simulink model "delay"  (R2025b)
settings: Solver=FixedStepDiscrete  StartTime=0.0  StopTime=inf  RelTol=1e-3
model workspace (MATLAB code in the model file):
  | Mix_rt = Simulink.Parameter(0.50);
  | Mix_rt.CoderInfo.StorageClass = 'Auto';   % <- NO ExportedGlobal
undefined symbols (not defined in the file): Mode_rt, Repeats_rt, Time_rt
settings Model: Creator=linogarciamorales  LastModifiedBy=linogarciamorales
settings OptimizationCC: EnhancedBackFolding=on  PassReuseOutputArgsAs=Individual arguments  ZeroExternalMemoryAtStartup=off  ZeroInternalMemoryAtStartup=off  OptimizeBlockOrder=speed  DifferentSizesBufferReuse=on  OptimizationCustomize=off  EfficientTunableParamExpr=on
settings DebuggingCC: ParameterTunabilityLossMsg=error
settings SFSimCC: MATLABDynamicMemAlloc=off
settings RTWCC: SystemTargetFile=ert.tlc  GenCodeOnly=on  TemplateMakefile=ert_default_tmf  Description=Embedded Coder
settings CodeAppCC: ForceParamTrailComments=on  IgnoreCustomStorageClasses=off  OperatorAnnotations=on  SimulinkDataObjDesc=on  SFDataObjDesc=on  InsertBlockDesc=on
settings ERTTargetCC: InlinedParameterPlacement=Hierarchical  ERTCustomFileTemplate=example_file_process.tlc  TargetLangStandard=C99 (ISO)  GenerateSampleERTMain=on  SupportNonInlinedSFcns=on

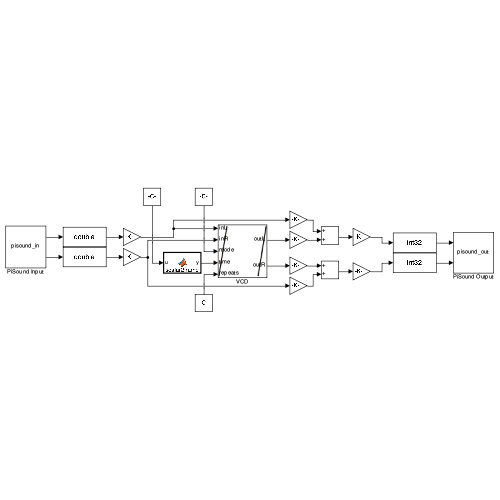
[thumbnail: Simulink's stored preview of the top-level diagram]
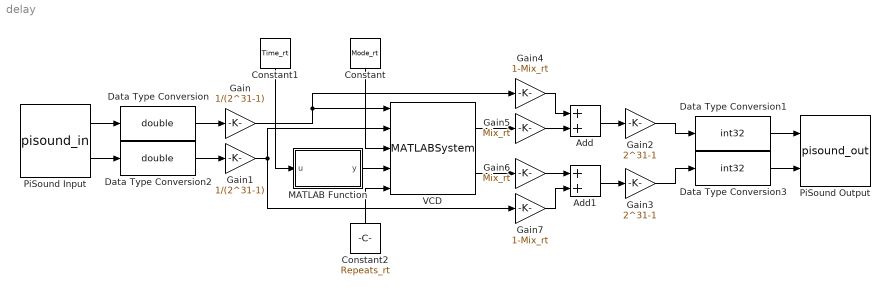
== system delay ==
  Add : Sum
  Add1 : Sum
  Constant : Constant  Value=Mode_rt  OutDataTypeStr=uint8
  Constant1 : Constant  Value=Time_rt  OutDataTypeStr=double
  Constant2 : Constant  Value=Repeats_rt  OutDataTypeStr=double
  Data Type Conversion : DataTypeConversion  OutDataTypeStr=double  SaturateOnIntegerOverflow=off  RndMeth=Floor
  Data Type Conversion1 : DataTypeConversion  OutDataTypeStr=int32  SaturateOnIntegerOverflow=off  RndMeth=Floor
  Data Type Conversion2 : DataTypeConversion  OutDataTypeStr=double  SaturateOnIntegerOverflow=off  RndMeth=Floor
  Data Type Conversion3 : DataTypeConversion  OutDataTypeStr=int32  SaturateOnIntegerOverflow=off  RndMeth=Floor
  Gain : Gain  Gain=1/(2^31-1)
  Gain1 : Gain  Gain=1/(2^31-1)
  Gain2 : Gain  Gain=2^31-1
  Gain3 : Gain  Gain=2^31-1
  Gain4 : Gain  Gain=1-Mix_rt  OutDataTypeStr=double
  Gain5 : Gain  Gain=Mix_rt  OutDataTypeStr=double
  Gain6 : Gain  Gain=Mix_rt  OutDataTypeStr=double
  Gain7 : Gain  Gain=1-Mix_rt  OutDataTypeStr=double
  MATLAB Function : MATLAB Function  TreatAsAtomicUnit=on
  PiSound Input : S-Function  FunctionName=pisound_in  Parameters=48000, 128, 0  SFunctionDeploymentMode=off  EnableBusSupport=off
  PiSound Output : S-Function  FunctionName=pisound_out  Parameters=48000, 128, 0  SFunctionDeploymentMode=off  EnableBusSupport=off
  VCD : MATLABSystem  System=vcd_sys  N=128  Fs=48000  MaxDelay=2  Mode=uint8(1)  Delay=0.1  g=0.5  SimulateUsing=Code generation
      mask Type: vcd_sys
  wires:
  PiSound Input/1 -> Data Type Conversion/1
  PiSound Input/2 -> Data Type Conversion2/1
  Data Type Conversion1/1 -> PiSound Output/1
  Data Type Conversion3/1 -> PiSound Output/2
  Gain2/1 -> Data Type Conversion1/1
  Gain3/1 -> Data Type Conversion3/1
  Data Type Conversion/1 -> Gain/1
  Data Type Conversion2/1 -> Gain1/1
  Gain/1 -> Gain4/1, VCD/1
  Gain1/1 -> Gain7/1, VCD/2
  VCD/1 -> Gain5/1
  VCD/2 -> Gain6/1
  Constant/1 -> VCD/3
  Constant2/1 -> VCD/5
  Add/1 -> Gain2/1
  Gain4/1 -> Add/1
  Gain5/1 -> Add/2
  Add1/1 -> Gain3/1
  Gain6/1 -> Add1/1
  Gain7/1 -> Add1/2
  MATLAB Function/1(y) -> VCD/4
  Constant1/1 -> MATLAB Function/1(u)

== matlab function delay/MATLAB Function ==
  data: u input; y output
function y = scalar2frame(u)
% u: escalar
% y: [N x 1]
N = 128;     % usa el mismo N del proyecto
y = u + zeros(N,1);
end
